simulink model "M9_ex2"  (R2022a)
settings: Solver=ode4  StartTime=0.0  StopTime=500  FixedStep=0.01  RelTol=1e-3
settings Model: Creator=hntran  LastModifiedBy=hntran

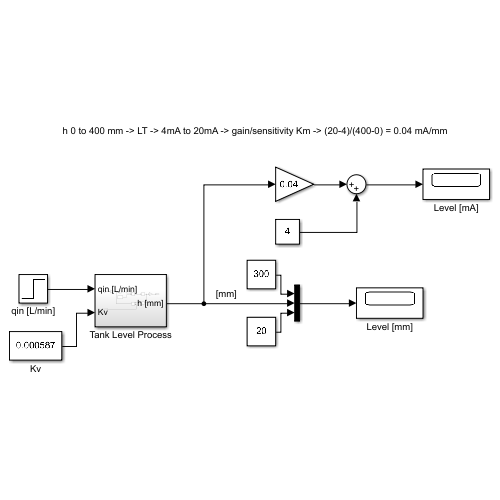
[thumbnail: Simulink's stored preview of the top-level diagram]
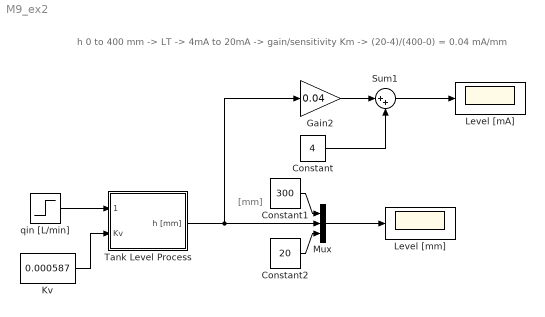
== system M9_ex2 ==
  note: h 0 to 400 mm -> LT -> 4mA to 20mA -> gain/sensitivity Km -> (20-4)/(400-0) = 0.04 mA/mm
  note: [mm]
  Constant : Constant  Value=4
  Constant1 : Constant  Value=300
  Constant2 : Constant  Value=20
  Gain2 : Gain  Gain=0.04
  Kv : Constant  Value=0.000587
  Level [mA] : Scope
  Level [mm] : Scope
  Mux : Mux  Inputs=3
  Sum1 : Sum  Inputs=|++
  Tank Level Process : Subsystem
  qin [L/min] : Step  Time=0  After=15  SampleTime=0
  wires:
  Constant/1 -> Sum1/2
  Gain2/1 -> Sum1/1
  Sum1/1 -> Level [mA]/1
  Constant1/1 -> Mux/1
  Constant2/1 -> Mux/3
  Mux/1 -> Level [mm]/1
  Tank Level Process/1(h [mm]) -> Gain2/1, Mux/2
  qin [L/min]/1 -> Tank Level Process/1(qin [L/min])
  Kv/1 -> Tank Level Process/2(Kv)

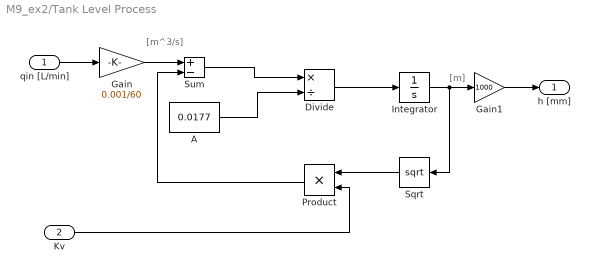
== system M9_ex2/Tank Level Process ==
  note: [m]
  note: [m^3/s]
  qin [L/min] : Inport
  Kv : Inport  Port=2
  A : Constant  Value=0.0177
  Divide : Product  Inputs=*/
  Gain : Gain  Gain=0.001/60
  Gain1 : Gain  Gain=1000
  Integrator : Integrator
  Product : Product
  Sqrt : Sqrt
  Sum : Sum  Inputs=+-
  h [mm] : Outport
  wires:
  Kv/1 -> Product/2
  Sqrt/1 -> Product/1
  Divide/1 -> Integrator/1
  Gain/1 -> Sum/1
  A/1 -> Divide/2
  Integrator/1 -> Gain1/1, Sqrt/1
  Product/1 -> Sum/2
  Sum/1 -> Divide/1
  qin [L/min]/1 -> Gain/1
  Gain1/1 -> h [mm]/1
